simulink model "PDU_Embedded_Implementation"  (R2024b)
settings: Solver=VariableStepAuto  StartTime=0.0  StopTime=15.0  RelTol=1e-3
libraries: spsVoltageMeasurementLib x4, spsSeriesRLCBranchLib x2, spsControlledVoltageSourceLib x2, spsGroundLib x2, spsIdealSwitchLib x2, msbAdcArchitectures x1, spspowerguiLib x1

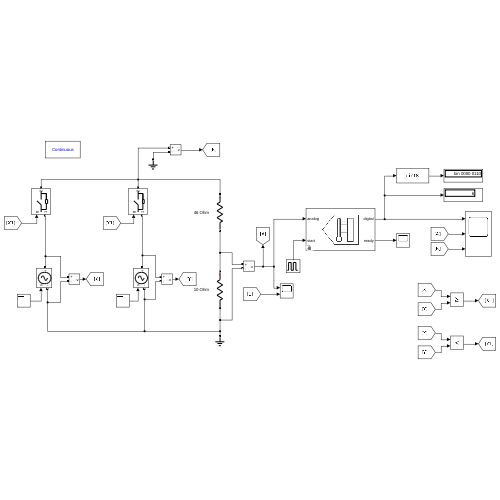
[thumbnail: Simulink's stored preview of the top-level diagram]
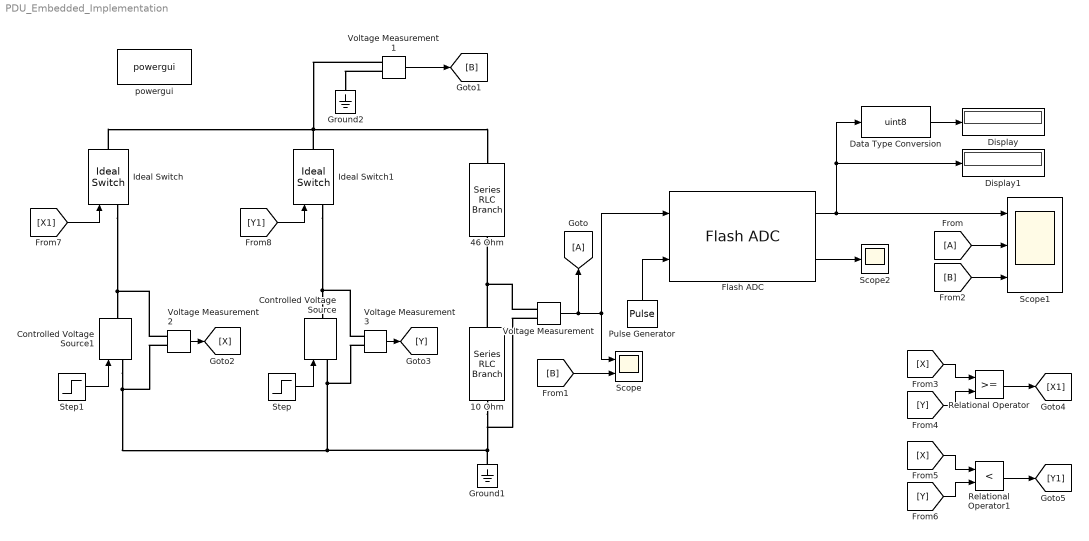
== system PDU_Embedded_Implementation ==
  10 Ohm : spsSeriesRLCBranchLib/Series RLC Branch  LConnTagsString=__new0  RConnTagsString=__new0  BranchType=R  Resistance=10  Inductance=1e-3  SetiL0=off  InitialCurrent=0  Capacitance=1e-6  Setx0=off  InitialVoltage=0  Measurements=None
  46 Ohm : spsSeriesRLCBranchLib/Series RLC Branch  LConnTagsString=__new0  RConnTagsString=__new0  BranchType=R  Resistance=46  Inductance=1e-3  SetiL0=off  InitialCurrent=0  Capacitance=1e-6  Setx0=off  InitialVoltage=0  Measurements=None
  Controlled Voltage Source : spsControlledVoltageSourceLib/Controlled Voltage Source  Initialize=on  Source_Type=DC  Amplitude=0  Phase=0  Frequency=0  Measurements=None
  Controlled Voltage Source1 : spsControlledVoltageSourceLib/Controlled Voltage Source  Initialize=on  Source_Type=DC  Amplitude=0  Phase=0  Frequency=0  Measurements=None
  Data Type Conversion : DataTypeConversion  OutDataTypeStr=uint8  SaturateOnIntegerOverflow=off  RndMeth=Floor
  Display : Display
      settings: Format=binary (Stored Integer)
  Display1 : Display
  Flash ADC : msbAdcArchitectures/Flash ADC  LabelModeActiveChoice=Simulink Blocks  NBits=4  InputRange=[0 5]  ExtStartClk=on  StartFreq=1e6  StartClkJitter=1e-12  SampleInterval=0.25e-6  Trigger=Rising edge  MatchScale=off  OutputPolarity=Auto  OutDataType=single  SimulateUsing=Simulink blocks  EnableLinearityImpairments=off  OffsetError=3  OffsetErrorUnit=LSB  GainError=2  GainErrorUnit=LSB  Bubbles=[]  EnableTimingImpairments=off  ConversionDelay=0  EnableIncreasedBufferSize=off  BufferSize=100
  From : From
  Goto : Goto
  Ground1 : spsGroundLib/Ground  LConnTagsString=a
  Ground2 : spsGroundLib/Ground  LConnTagsString=a
  Ideal Switch : spsIdealSwitchLib/Ideal Switch  Ron=0.001  Lon=0  IC=0  Rs=1e5  Cs=inf  Measurements=off
  Ideal Switch1 : spsIdealSwitchLib/Ideal Switch  Ron=0.001  Lon=0  IC=0  Rs=1e5  Cs=inf  Measurements=off
  Pulse Generator : DiscretePulseGenerator  PulseType=Time based  Period=0.0001  PulseWidth=50
  Relational Operator : RelationalOperator  OutDataTypeStr=boolean  RndMeth=Simplest  InputSameDT=off
  Relational Operator1 : RelationalOperator  Operator=<  OutDataTypeStr=boolean  RndMeth=Simplest  InputSameDT=off
  Scope : Scope  NumInputPorts=2
  Scope1 : Scope  NumInputPorts=3
  Scope2 : Scope
  Step : Step  Time=4  Before=28  After=10  SampleTime=0
  Step1 : Step  Time=8  Before=25  After=10  SampleTime=0
  Voltage Measurement{,1..3} (4 alike) : spsVoltageMeasurementLib/Voltage Measurement  PhasorSimulation=off  OutputType=Complex  PSBequivalent=0
  powergui : spspowerguiLib/powergui  Priority=1  SimulationMode=Continuous  SampleTime=50e-6  frequency=60  Iterations=50  frequencyindice=0  Pbase=100e6  ErrMax=1e-4  UnitsV=kV  UnitsW=MW  buscounter=0  FunctionMessages=off  echomessages=off  EnableUseOfTLC=off  CurrentSourceSwitches=off  DisableSnubberDevices=off  DisableRonSwitches=off  DisableVfSwitches=off  DisplayEquations=off  AutomaticDiscreteSolvers=off  SolverType=Tustin/Backward Euler (TBE)  Interpol=off  ExternalGateDelay=off  methode=off  Ts=100  x0status=blocks  SPID=on  SwTol=0  HookPort=off  NonlinearTolerance=1e-4  nMaxIteration=100  ContinueOnMaxIteration=off  RestoreLinks=warning  ResistiveCurrentMeasurement=off  Frange=[0:2:500]  Ylog=off  Xlog=on  ShowGrid=off  save=off  variable=ZData  structure=0  ZoomFFT=off  StartTime=0.0  cycles=1  DisplayStyle=1  fundamental=60  FreqAxis=off  MaxFrequency=1000  frequencyindicesteady=1  RmsSteady=1  display=off
  wires:
  Voltage Measurement/1 -> Goto/1, Flash ADC/1, Scope/1
  Step/1 -> Controlled Voltage Source/1
  Step1/1 -> Controlled Voltage Source1/1
  Flash ADC/1 -> Display1/1, Data Type Conversion/1, Scope1/1
  Flash ADC/2 -> Scope2/1
  Pulse Generator/1 -> Flash ADC/2
  Data Type Conversion/1 -> Display/1
  Voltage Measurement1/1 -> [B]
  From/1 -> Scope1/2
  [B] -> Scope/2
  [B] -> Scope1/3
  Voltage Measurement2/1 -> [X]
  Voltage Measurement3/1 -> [Y]
  [X] -> Relational Operator/1
  [Y] -> Relational Operator/2
  Relational Operator/1 -> [X1]
  [X] -> Relational Operator1/1
  [Y] -> Relational Operator1/2
  Relational Operator1/1 -> [Y1]
  [X1] -> Ideal Switch/1
  [Y1] -> Ideal Switch1/1
  connections:
  Voltage Measurement/LConn1 -- 46 Ohm/RConn1 -- 10 Ohm/LConn1
  Controlled Voltage Source1/LConn1 -- Voltage Measurement2/LConn2 -- 10 Ohm/RConn1 -- Voltage Measurement/LConn2 -- Ground1/LConn1 -- Controlled Voltage Source/LConn1 -- Voltage Measurement3/LConn2
  Ideal Switch1/LConn1 -- Voltage Measurement3/LConn1 -- Controlled Voltage Source/RConn1
  Ideal Switch/LConn1 -- Voltage Measurement2/LConn1 -- Controlled Voltage Source1/RConn1
  Voltage Measurement1/LConn1 -- Ideal Switch/RConn1 -- Ideal Switch1/RConn1 -- 46 Ohm/LConn1
  Voltage Measurement1/LConn2 -- Ground2/LConn1
